simulink model "Motor_Poition"  (R2020a)
settings: Solver=VariableStepAuto  StartTime=0.0  StopTime=120.0  RelTol=1e-3
undefined symbols (not defined in the file or in its folder): b, J, K, L, R
settings Model: DataDictionary=DcMotorData.sldd  Creator=kasutav  LastModifiedBy=kasutav
settings DataIOCC: SaveOutput=off  SaveTime=off

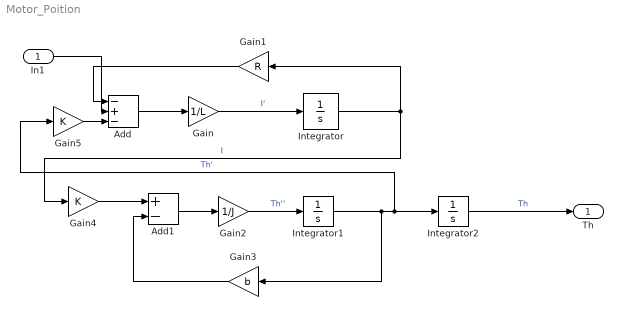
== system Motor_Poition ==
  In1 : Inport  OutDataTypeStr=double  PortDimensions=1  SampleTime=0
  Add : Sum  Inputs=-+-
  Add1 : Sum  Inputs=+-
  Gain : Gain  Gain=1/L
  Gain1 : Gain  Gain=R
  Gain2 : Gain  Gain=1/J
  Gain3 : Gain  Gain=b
  Gain4 : Gain  Gain=K
  Gain5 : Gain  Gain=K
  Integrator : Integrator
  Integrator1 : Integrator
  Integrator2 : Integrator
  Th : Outport  OutDataTypeStr=double  PortDimensions=1  SampleTime=0
  wires:
  Gain1/1 -> Add/1
  Add/1 -> Gain/1
  Add1/1 -> Gain2/1
  In1/1 -> Add/2
  Integrator/1 -> Gain1/1, Gain4/1  "I"
  Integrator1/1 -> Integrator2/1, Gain5/1, Gain3/1  "Th'"
  Integrator2/1 -> Th/1  "Th"
  Gain/1 -> Integrator/1  "I'"
  Gain2/1 -> Integrator1/1  "Th''"
  Gain4/1 -> Add1/1
  Gain5/1 -> Add/3
  Gain3/1 -> Add1/2
